simulink model "punto8"  (R2015a)
settings: Solver=ode45  StartTime=0.0  StopTime=10.0  RelTol=1e-3
settings Model: Creator=Administrador  LastModifiedBy=Administrador

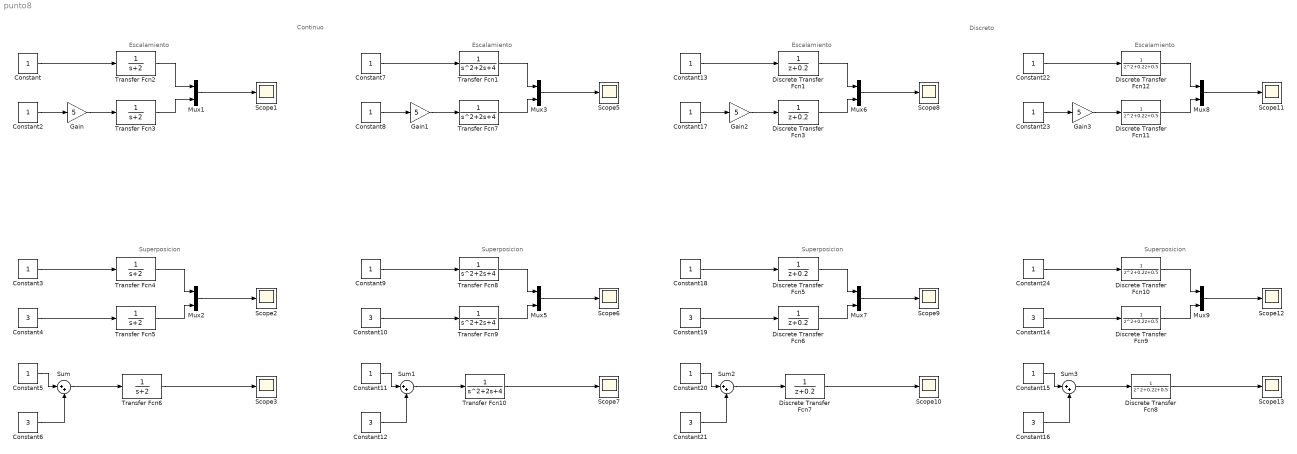
== system punto8 ==
  note: Continuo
  note: Discreto
  note: Superposicion
  note: Escalamiento
  note: Superposicion
  note: Escalamiento
  note: Superposicion
  note: Escalamiento
  note: Superposicion
  note: Escalamiento
  Constant{,2..3,5,7..9,11,13,15,17..18,20,22..24} (16 alike) : Constant
  Constant{4,6,10,12,14,16,19,21} (8 alike) : Constant  Value=3
  Discrete Transfer Fcn{1,3,5..7} (5 alike) : DiscreteTransferFcn  Denominator=[1 0.2]  SampleTime=0.1
  Discrete Transfer Fcn{8..12} (5 alike) : DiscreteTransferFcn  Denominator=[1 0.2 0.5]  SampleTime=0.1
  Gain{,1..3} (4 alike) : Gain  Gain=5
  Mux{1..3,5..9} (8 alike) : Mux  Inputs=2
  Scope{1..3,5..13} (12 alike) : Scope
      Scope10 settings: SaveName=ScopeData7
      Scope11 settings: SaveName=ScopeData8
      Scope12 settings: SaveName=ScopeData9
      Scope13 settings: SaveName=ScopeData10
      Scope3 settings: SaveName=ScopeData2
      Scope5 settings: SaveName=ScopeData3
      Scope6 settings: SaveName=ScopeData5
      Scope7 settings: SaveName=ScopeData6
      Scope8 settings: SaveName=ScopeData11
      Scope9 settings: SaveName=ScopeData12
  Sum{,1..3} (4 alike) : Sum  Inputs=|++
  Transfer Fcn{1,7..10} (5 alike) : TransferFcn  Denominator=[1 2 4]
  Transfer Fcn{2..6} (5 alike) : TransferFcn  Denominator=[1 2]
  wires:
  Constant/1 -> Transfer Fcn2/1
  Constant2/1 -> Gain/1
  Gain/1 -> Transfer Fcn3/1
  Mux1/1 -> Scope1/1
  Transfer Fcn2/1 -> Mux1/1
  Transfer Fcn3/1 -> Mux1/2
  Constant3/1 -> Transfer Fcn4/1
  Constant4/1 -> Transfer Fcn5/1
  Mux2/1 -> Scope2/1
  Transfer Fcn4/1 -> Mux2/1
  Transfer Fcn5/1 -> Mux2/2
  Constant5/1 -> Sum/1
  Constant6/1 -> Sum/2
  Sum/1 -> Transfer Fcn6/1
  Transfer Fcn6/1 -> Scope3/1
  Constant7/1 -> Transfer Fcn1/1
  Constant8/1 -> Gain1/1
  Gain1/1 -> Transfer Fcn7/1
  Mux3/1 -> Scope5/1
  Transfer Fcn1/1 -> Mux3/1
  Transfer Fcn7/1 -> Mux3/2
  Constant9/1 -> Transfer Fcn8/1
  Constant10/1 -> Transfer Fcn9/1
  Mux5/1 -> Scope6/1
  Transfer Fcn8/1 -> Mux5/1
  Transfer Fcn9/1 -> Mux5/2
  Constant11/1 -> Sum1/1
  Constant12/1 -> Sum1/2
  Sum1/1 -> Transfer Fcn10/1
  Transfer Fcn10/1 -> Scope7/1
  Constant13/1 -> Discrete Transfer Fcn1/1
  Constant17/1 -> Gain2/1
  Gain2/1 -> Discrete Transfer Fcn3/1
  Mux6/1 -> Scope8/1
  Discrete Transfer Fcn1/1 -> Mux6/1
  Discrete Transfer Fcn3/1 -> Mux6/2
  Constant18/1 -> Discrete Transfer Fcn5/1
  Constant19/1 -> Discrete Transfer Fcn6/1
  Mux7/1 -> Scope9/1
  Discrete Transfer Fcn5/1 -> Mux7/1
  Discrete Transfer Fcn6/1 -> Mux7/2
  Constant20/1 -> Sum2/1
  Constant21/1 -> Sum2/2
  Sum2/1 -> Discrete Transfer Fcn7/1
  Discrete Transfer Fcn7/1 -> Scope10/1
  Constant22/1 -> Discrete Transfer Fcn12/1
  Constant23/1 -> Gain3/1
  Gain3/1 -> Discrete Transfer Fcn11/1
  Mux8/1 -> Scope11/1
  Discrete Transfer Fcn12/1 -> Mux8/1
  Discrete Transfer Fcn11/1 -> Mux8/2
  Constant24/1 -> Discrete Transfer Fcn10/1
  Constant14/1 -> Discrete Transfer Fcn9/1
  Mux9/1 -> Scope12/1
  Discrete Transfer Fcn10/1 -> Mux9/1
  Discrete Transfer Fcn9/1 -> Mux9/2
  Constant15/1 -> Sum3/1
  Constant16/1 -> Sum3/2
  Sum3/1 -> Discrete Transfer Fcn8/1
  Discrete Transfer Fcn8/1 -> Scope13/1
